simulink model "fuselage_th"  (R2018b)
settings: Solver=VariableStepAuto  StartTime=0.0  StopTime=10.0  RelTol=1e-3
libraries: fuselage_cl x1
settings Model: Creator=jldanie5  LastModifiedBy=jldanie5

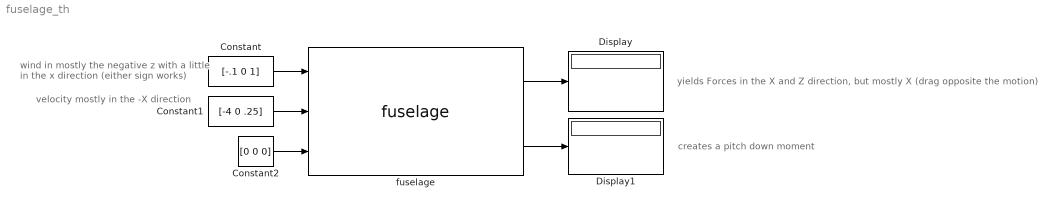
== system fuselage_th ==
  note: creates a pitch down moment
  note: yields Forces in the X and Z direction, but mostly X (drag opposite the motion)
  note: velocity mostly in the -X direction
  note: wind in mostly the negative z with a little
      |  in the x direction (either sign works)
  Constant : Constant  Value=[-.1 0 1]
  Constant1 : Constant  Value=[-4 0 .25]
  Constant2 : Constant  Value=[0 0 0]
  Display : Display
  Display1 : Display
  fuselage : fuselage_cl/fuselage  fus=vhcl.fuse  fusRhoDa=env.water.density.Value
  wires:
  Constant/1 -> fuselage/1
  Constant1/1 -> fuselage/2
  Constant2/1 -> fuselage/3
  fuselage/1 -> Display/1
  fuselage/2 -> Display1/1
